simulink model "CANBlocksTemplate"  (Simulink 10.0)
settings: Solver=ode45  StartTime=0.0  StopTime=10.0  RelTol=1e-3  EnableMultiTasking=on
undefined symbols (not defined in the file): IO_Blk_Lib_TTC500, IO_Blk_Lib_TTC9094, IO_CAN_ConfigMsg, IO_CAN_Init, IO_CAN_ReadMsg
libraries: simulink x19, IOBlock_Library_TTC580 x18
(part 1 of 2)
settings Model: Creator=hokka  LastModifiedBy=hokka
settings Model: SuppressorTable=|
  | <?xml version="1.0" encoding="UTF-8" standalone="yes" ?>
  | <!DOCTYPE boost_serialization>
  | <boost_serialization signature="serialization::archive" version="15">
  | <DiagnosticSuppressor class_id="0" tracking_level="0" version="6">
  | 	<Table class_id="1" tracking_level="0" version="0">
  | 		<count>8</count>
  | 		<bucket_count>8</bucket_count>
  | 		<item_version>0</item_version>
  | 		<item class_id="2" tracking_level="0" version="0">
  | 			<first class_id="3" tracking_level="0" version="6">
  | 				<Source class_id="4" tracking_level="0" version="0">
  | 					<count>1</count>
  | 					<item_version>0</item_version>
  | 					<item>CANBlocksTemplate/CAN_RX_ND/Trigger_Block/Counter Limited</item>
  | 				</Source>
  | 			</first>
  | 			<second class_id="5" tracking_level="0" version="6">
  | 				<SuppressedData class_id="6" tracking_level="0" version="0">
  | 					<count>2</count>
  | 					<bucket_count>8</bucket_count>
  | 					<item_version>0</item_version>
  | 					<item class_id="7" tracking_level="0" version="0">
  | 						<first class_id="8" tracking_level="0" version="6">
  | 							<ID>SimulinkFixedPoint:util:Overflowoccurred</ID>
  | 							<Cause>
  | 								<Source>
  | 									<count>0</count>
  | 									<item_version>0</item_version>
  | 								</Source>
  | 							</Cause>
  | 						</first>
  | 						<second class_id="9" tracking_level="0" version="6">
  | 							<Comment></Comment>
  | 							<User></User>
  | 							<LastModified class_id="10" tracking_level="0" version="0">
  | 								<ptime_date class_id="11" tracking_level="0" version="0">
  | 									<date>20160608</date>
  | 								</ptime_date>
  | 								<ptime_time_duration class_id="12" tracking_level="0" version="0">
  | 									<is_special>0</is_special>
  | 									<time_duration_hours>15</time_duration_hours>
  | 									<time_duration_minutes>23</time_duration_minutes>
  | 									<time_duration_seconds>17</time_duration_seconds>
  | 									<time_duration_fractional_seconds>0</time_duration_fractional_seconds>
  | 								</ptime_time_duration>
  | 							</LastModified>
  | 							<SuppressionType>1</SuppressionType>
  | 						</second>
  | 					</item>
  | 					<item>
  | 						<first>
  | 							<ID>Simulink:DataType:WarningOverFlowDetected</ID>
  | 							<Cause>
  | 								<Source>
  | 									<count>0</count>
  | 									<item_version>0</item_version>
  | 								</Source>
  | 							</Cause>
  | 						</first>
  | 						<second>
  | 							<Comment></Comment>
  | 							<User></User>
  | 							<LastModified>
  | 								<ptime_date>
  | 									<date>20160608</date>
  | 								</ptime_date>
  | 								<ptime_time_duration>
  | 									<is_special>0</is_special>
  | 									<time_duration_hours>15</time_duration_hours>
  | 									<time_duration_minutes>23</time_duration_minutes>
  | 									<time_duration_seconds>17</time_duration_seconds>
  | 									<time_duration_fractional_seconds>0</time_duration_fractional_seconds>
  | 								</ptime_time_duration>
  | 							</LastModified>
  | 							<SuppressionType>1</SuppressionType>
  | 						</second>
  | 					</item>
  | 				</SuppressedData>
  | 			</second>
  | 		</item>
  | 		<item>
  | 			<first>
  | 				<Source>
  | 					<count>1</count>
  | 					<item_version>0</item_version>
  | 					<item>CANBlocksTemplate/CAN_TX/Trigger_Block/Counter Limited</item>
  | 				</Source>
  | 			</first>
  | 			<second>
  | 				<SuppressedData>
  | 					<count>2</count>
  | 					<bucket_count>8</bucket_count>
  | 					<item_version>0</item_version>
  | 					<item>
  | 						<first>
  | 							<ID>SimulinkFixedPoint:util:Overflowoccurred</ID>
  | 							<Cause>
  | 								<Source>
  | 									<count>0</count>
  | 									<item_version>0</item_version>
  | 								</Source>
  | 							</Cause>
  | 						</first>
  | 						<second>
  | 							<Comment></Comment>
  | 							<User></User>
  | 							<LastModified>
  | 								<ptime_date>
  | 									<date>20160608</date>
  | 								</ptime_date>
  | 								<ptime_time_duration>
  | 									<is_special>0</is_special>
  | 									<time_duration_hours>15</time_duration_hours>
  | 									<time_duration_minutes>23</time_duration_minutes>
  | 									<time_duration_seconds>17</time_duration_seconds>
  | 									<time_duration_fractional_seconds>0</time_duration_fractional_seconds>
  | 								</ptime_time_duration>
  | 							</LastModified>
  | 							<SuppressionType>1</SuppressionType>
  | 						</second>
  | 					</item>
  | 					<item>
  | 						<first>
  | 							<ID>Simulink:DataType:WarningOverFlowDetected</ID>
  | 							<Cause>
  | 								<Source>
  | 									<count>0</count>
  | 									<item_version>0</item_version>
  | 								</Source>
  | 							</Cause>
  | 						</first>
  | 						<second>
  | 							<Comment></Comment>
  | 							<User></User>
  | 							<LastModified>
  | 								<ptime_date>
  | 									<date>20160608</date>
  | 								</ptime_date>
  | 								<ptime_time_duration>
  | 									<is_special>0</is_special>
  | 									<time_duration_hours>15</time_duration_hours>
  | 									<time_duration_minutes>23</time_duration_minutes>
  | 									<time_duration_seconds>17</time_duration_seconds>
  | 									<time_duration_fractional_seconds>0</time_duration_fractional_seconds>
  | 								</ptime_time_duration>
  | 							</LastModified>
  | 							<SuppressionType>1</SuppressionType>
  | 						</second>
  | 					</item>
  | 				</SuppressedData>
  | 			</second>
  | 		</item>
  | 		<item>
  | 			<first>
  | 				<Source>
  | 					<count>1</count>
  | 					<item_version>0</item_version>
  | 					<item>CANBlocksTemplate/CAN_RX_NONE_ND/Trigger_Block/Counter Limited</item>
  | 				</Source>
  | 			</first>
  | 			<second>
  | 				<SuppressedData>
  | 					<count>2</count>
  | 					<bucket_count>8</bucket_count>
  | 					<item_version>0</item_version>
  | 					<item>
  | 						<first>
  | 							<ID>SimulinkFixedPoint:util:Overflowoccurred</ID>
  | 							<Cause>
  | 								<Source>
  | 									<count>0</count>
  | 									<item_version>0</item_version>
  | 								</Source>
  | 							</Cause>
  | 						</first>
  | 						<second>
  | 							<Comment></Comment>
  | 							<User></User>
  | 							<LastModified>
  | 								<ptime_date>
  | 									<date>20160608</date>
  | 								</ptime_date>
  | 								<ptime_time_duration>
  | 									<is_special>0</is_special>
  | 									<time_duration_hours>15</time_duration_hours>
  | 									<time_duration_minutes>23</time_duration_minutes>
  | 									<time_duration_seconds>17</time_duration_seconds>
  | 									<time_duration_fractional_seconds>0</time_duration_fractional_seconds>
  | 								</ptime_time_duration>
  | 							</LastModified>
  | 							<SuppressionType>1</SuppressionType>
  | 						</second>
  | 					</item>
  | 					<item>
  | 						<first>
  | 							<ID>Simulink:DataType:WarningOverFlowDetected</ID>
  | 							<Cause>
  | 								<Source>
  | 									<count>0</count>
  | 									<item_version>0</item_version>
  | 								</Source>
  | 							</Cause>
  | 						</first>
  | 						<second>
  | 							<Comment></Comment>
  | 							<User></User>
  | 							<LastModified>
  | 								<ptime_date>
  | 									<date>20160608</date>
  | 								</ptime_date>
  | 								<ptime_time_duration>
  | 									<is_special>0</is_special>
  | 									<time_duration_hours>15</time_duration_hours>
  | 									<time_duration_minutes>23</time_duration_minutes>
  | 									<time_duration_seconds>17</time_duration_seconds>
  | 									<time_duration_fractional_seconds>0</time_duration_fractional_seconds>
  | 								</ptime_time_duration>
  | 							</LastModified>
  | 							<SuppressionType>1</SuppressionType>
  | 						</second>
  | 					</item>
  | 				</SuppressedData>
  | 			</second>
  | 		</item>
  | 		<item>
  | 			<first>
  | 				<Source>
  | 					<count>1</count>
  | 					<item_version>0</item_version>
  | 					<item>CANBlocksTemplate/CAN_TX_NONE_aggr/Trigger_Block/Counter Limited</item>
  | 				</Source>
  | 			</first>
  | 			<second>
  | 				<SuppressedData>
  | 					<count>2</count>
  | 					<bucket_count>8</bucket_count>
  | 					<item_version>0</item_version>
  | 					<item>
  | 						<first>
  | 							<ID>SimulinkFixedPoint:util:Overflowoccurred</ID>
  | 							<Cause>
  | 								<Source>
  | 									<count>0</count>
  | 									<item_version>0</item_version>
  | 								</Source>
  | 							</Cause>
  | 						</first>
  | 						<second>
  | 							<Comment></Comment>
  | 							<User></User>
  | 							<LastModified>
  | 								<ptime_date>
  | 									<date>20160608</date>
  | 								</ptime_date>
  | 								<ptime_time_duration>
  | 									<is_special>0</is_special>
  | 									<time_duration_hours>15</time_duration_hours>
  | 									<time_duration_minutes>23</time_duration_minutes>
  | 									<time_duration_seconds>17</time_duration_seconds>
  | 									<time_duration_fractional_seconds>0</time_duration_fractional_seconds>
  | 								</ptime_time_duration>
  | 							</LastModified>
  | 							<SuppressionType>1</SuppressionType>
  | 						</second>
  | 					</item>
  | 					<item>
  | 						<first>
  | 							<ID>Simulink:DataType:WarningOverFlowDetected</ID>
  | 							<Cause>
  | 								<Source>
  | 									<count>0</count>
  | 									<item_version>0</item_version>
  | 								</Source>
  | 							</Cause>
  | 						</first>
  | 						<second>
  | 							<Comment></Comment>
  | 							<User></User>
  | 							<LastModified>
  | 								<ptime_date>
  | 									<date>20160608</date>
  | 								</ptime_date>
  | 								<ptime_time_duration>
  | 									<is_special>0</is_special>
  | 									<time_duration_hours>15</time_duration_hours>
  | 									<time_duration_minutes>23</time_duration_minutes>
  | 									<time_duration_seconds>17</time_duration_seconds>
  | 									<time_duration_fractional_seconds>0</time_duration_fractional_seconds>
  | 								</ptime_time_duration>
  | 							</LastModified>
  | 							<SuppressionType>1</SuppressionType>
  | 						</second>
  | 					</item>
  | 				</SuppressedData>
  | 			</second>
  | 		</item>
  | 		<item>
  | 			<first>
  | 				<Source>
  | 					<count>1</count>
  | 					<item_version>0</item_version>
  | 					<item>CANBlocksTemplate/CAN_TX_NONE/Trigger_Block/Counter Limited</item>
  | 				</Source>
  | 			</first>
  | 			<second>
  | 				<SuppressedData>
  | 					<count>2</count>
  | 					<bucket_count>8</bucket_count>
  | 					<item_version>0</item_version>
  | 					<item>
  | 						<first>
  | 							<ID>SimulinkFixedPoint:util:Overflowoccurred</ID>
  | 							<Cause>
  | 								<Source>
  | 									<count>0</count>
  | 									<item_version>0</item_version>
  | 								</Source>
  | 							</Cause>
  | 						</first>
  | 						<second>
  | 							<Comment></Comment>
  | 							<User></User>
  | 							<LastModified>
  | 								<ptime_date>
  | 									<date>20160608</date>
  | 								</ptime_date>
  | 								<ptime_time_duration>
  | 									<is_special>0</is_special>
  | 									<time_duration_hours>15</time_duration_hours>
  | 									<time_duration_minutes>23</time_duration_minutes>
  | 									<time_duration_seconds>17</time_duration_seconds>
  | 									<time_duration_fractional_seconds>0</time_duration_fractional_seconds>
  | 								</ptime_time_duration>
  | 							</LastModified>
  | 							<SuppressionType>1</SuppressionType>
  | 						</second>
  | 					</item>
  | 					<item>
  | 						<first>
  | 							<ID>Simulink:DataType:WarningOverFlowDetected</ID>
  | 							<Cause>
  | 								<Source>
  | 									<count>0</count>
  | 									<item_version>0</item_version>
  | 								</Source>
  | 							</Cause>
  | 						</first>
  | 						<second>
  | 							<Comment></Comment>
  | 							<User></User>
  | 							<LastModified>
  | 								<ptime_date>
  | 									<date>20160608</date>
  | 								</ptime_date>
  | 								<ptime_time_duration>
  | 									<is_special>0</is_special>
  | 									<time_duration_hours>15</time_duration_hours>
  | 									<time_duration_minutes>23</time_duration_minutes>
  | 									<time_duration_seconds>17</time_duration_seconds>
  | 									<time_duration_fractional_seconds>0</time_duration_fractional_seconds>
  | 								</ptime_time_duration>
  | 							</LastModified>
  | 							<SuppressionType>1</SuppressionType>
  | 						</second>
  | 					</item>
  | 				</SuppressedData>
  | 			</second>
  | 		</item>
  | 		<item>
  | 			<first>
  | 				<Source>
  | 					<count>1</count>
  | 					<item_version>0</item_version>
  | 					<item>CANBlocksTemplate/CAN_RX/Trigger_Block/Counter Limited</item>
  | 				</Source>
  | 			</first>
  | 			<second>
  | 				<SuppressedData>
  | 					<count>2</count>
  | 					<bucket_count>8</bucket_count>
  | 					<item_version>0</item_version>
  | 					<item>
  | 						<first>
  | 							<ID>SimulinkFixedPoint:util:Overflowoccurred</ID>
  | 							<Cause>
  | 								<Source>
  | 									<count>0</count>
  | 									<item_version>0</item_version>
  | 								</Source>
  | 							</Cause>
  | 						</first>
  | 						<second>
  | 							<Comment></Comment>
  | 							<User></User>
  | 							<LastModified>
  | 								<ptime_date>
  | 									<date>20160608</date>
  | 								</ptime_date>
  | 								<ptime_time_duration>
  | 									<is_special>0</is_special>
  | 									<time_duration_hours>15</time_duration_hours>
  | 									<time_duration_minutes>23</time_duration_minutes>
  | 									<time_duration_seconds>17</time_duration_seconds>
  | 									<time_duration_fractional_seconds>0</time_duration_fractional_seconds>
  | 								</ptime_time_duration>
  | 							</LastModified>
  | 							<SuppressionType>1</SuppressionType>
  | 						</second>
  | 					</item>
  | 					<item>
  | 						<first>
  | 							<ID>Simulink:DataType:WarningOverFlowDetected</ID>
  | 							<Cause>
  | 								<Source>
  | 									<count>0</count>
  | 									<item_version>0</item_version>
  | 								</Source>
  | 							</Cause>
  | 						</first>
  | 						<second>
  | 							<Comment></Comment>
  | 							<User></User>
  | 							<LastModified>
  | 								<ptime_date>
  | 									<date>20160608</date>
  | 								</ptime_date>
  | 								<ptime_time_duration>
  | 									<is_special>0</is_special>
  | 									<time_duration_hours>15</time_duration_hours>
  | 									<time_duration_minutes>23</time_duration_minutes>
  | 									<time_duration_seconds>17</time_duration_seconds>
  | 									<time_duration_fractional_seconds>0</time_duration_fractional_seconds>
  | 								</ptime_time_duration>
  | 							</LastModified>
  | 							<SuppressionType>1</SuppressionType>
  | 						</second>
  | 					</item>
  | 				</SuppressedData>
  | 			</second>
  | 		</item>
  | 		<item>
  | 			<first>
  | 				<Source>
  | 					<count>1</count>
  | 					<item_version>0</item_version>
  | 					<item>CANBlocksTemplate/CAN_RX_NONE/Trigger_Block/Counter Limited</item>
  | 				</Source>
  | 			</first>
  | 			<second>
  | 				<SuppressedData>
  | 					<count>2</count>
  | 					<bucket_count>8</bucket_count>
  | 					<item_version>0</item_version>
  | 					<item>
  | 						<first>
  | 							<ID>SimulinkFixedPoint:util:Overflowoccurred</ID>
  | 							<Cause>
  | 								<Source>
  | 									<count>0</count>
  | 									<item_version>0</item_version>
  | 								</Source>
  | 							</Cause>
  | 						</first>
  | 						<second>
  | 							<Comment></Comment>
  | 							<User></User>
  | 							<LastModified>
  | 								<ptime_date>
  | 									<date>20160608</date>
  | 								</ptime_date>
  | 								<ptime_time_duration>
  | 									<is_special>0</is_special>
  | 									<time_duration_hours>15</time_duration_hours>
  | 									<time_duration_minutes>23</time_duration_minutes>
  | 									<time_duration_seconds>17</time_duration_seconds>
  | 									<time_duration_fractional_seconds>0</time_duration_fractional_seconds>
  | 								</ptime_time_duration>
  | 							</LastModified>
  | 							<SuppressionType>1</SuppressionType>
  | 						</second>
  | 					</item>
  | 					<item>
  | 						<first>
  | 							<ID>Simulink:DataType:WarningOverFlowDetected</ID>
  | 							<Cause>
  | 								<Source>
  | 									<count>0</count>
  | 									<item_version>0</item_version>
  | 								</Source>
  | 							</Cause>
  | 						</first>
  | 						<second>
  | 							<Comment></Comment>
  | 							<User></User>
  | 							<LastModified>
  | 								<ptime_date>
  | 									<date>20160608</date>
  | 								</ptime_date>
  | 								<ptime_time_duration>
  | 									<is_special>0</is_special>
  | 									<time_duration_hours>15</time_duration_hours>
  | 									<time_duration_minutes>23</time_duration_minutes>
  | 									<time_duration_seconds>17</time_duration_seconds>
  | 									<time_duration_fractional_seconds>0</time_duration_fractional_seconds>
  | 								</ptime_time_duration>
  | 							</LastModified>
  | 							<SuppressionType>1</SuppressionType>
  | 						</second>
  | 					</item>
  | 				</SuppressedData>
  | 			</second>
  | 		</item>
  | 		<item>
  | 			<first>
  | 				<Source>
  | 					<count>1</count>
  | 					<item_version>0</item_version>
  | 					<item>CANBlocksTemplate/CAN_TX_aggr/Trigger_Block/Counter Limited</item>
  | 				</Source>
  | 			</first>
  | 			<second>
  | 				<SuppressedData>
  | 					<count>2</count>
  | 					<bucket_count>8</bucket_count>
  | 					<item_version>0</item_version>
  | 					<item>
  | 						<first>
  | 							<ID>Simulink:DataType:WarningOverFlowDetected</ID>
  | 							<Cause>
  | 								<Source>
  | 									<count>0</count>
  | 									<item_version>0</item_version>
  | 								</Source>
  | 							</Cause>
  | 						</first>
  | 						<second>
  | 							<Comment></Comment>
  | 							<User></User>
  | 							<LastModified>
  | 								<ptime_date>
  | 									<date>20160608</date>
  | 								</ptime_date>
  | 								<ptime_time_duration>
  | 									<is_special>0</is_special>
  | 									<time_duration_hours>15</time_duration_hours>
  | 									<time_duration_minutes>23</time_duration_minutes>
  | 									<time_duration_seconds>17</time_duration_seconds>
  | 									<time_duration_fractional_seconds>0</time_duration_fractional_seconds>
  | 								</ptime_time_duration>
  | 							</LastModified>
  | 							<SuppressionType>1</SuppressionType>
  | 						</second>
  | 					</item>
  | 					<item>
  | 						<first>
  | 							<ID>SimulinkFixedPoint:util:Overflowoccurred</ID>
  | 							<Cause>
  | 								<Source>
  | 									<count>0</count>
  | 									<item_version>0</item_version>
  | 								</Source>
  | 							</Cause>
  | 						</first>
  | 						<second>
  | 							<Comment></Comment>
  | 							<User></User>
  | 							<LastModified>
  | 								<ptime_date>
  | 									<date>20160608</date>
  | 								</ptime_date>
  | 								<ptime_time_duration>
  | 									<is_special>0</is_special>
  | 									<time_duration_hours>15</time_duration_hours>
  | 									<time_duration_minutes>23</time_duration_minutes>
  | 									<time_duration_seconds>17</time_duration_seconds>
  | 									<time_duration_fractional_seconds>0</time_duration_fractional_seconds>
  | 								</ptime_time_duration>
  | 							</LastModified>
  | 							<SuppressionType>1</SuppressionType>
  | 						</second>
  | 					</item>
  | 				</SuppressedData>
  | 			</second>
  | 		</item>
  | 	</Table>
  | </DiagnosticSuppressor>
  | </boost_serialization>
settings DataIOCC: LimitDataPoints=on  SignalLoggingSaveFormat=ModelDataLogs
settings OptimizationCC: ExpressionDepthLimit=2147483647
settings DebuggingCC: SolverPrmCheckMsg=warning  FcnCallInpInsideContextMsg=warning  StateNameClashWarn=warning
settings ConfigComp: CovExternalEMLEnable=off

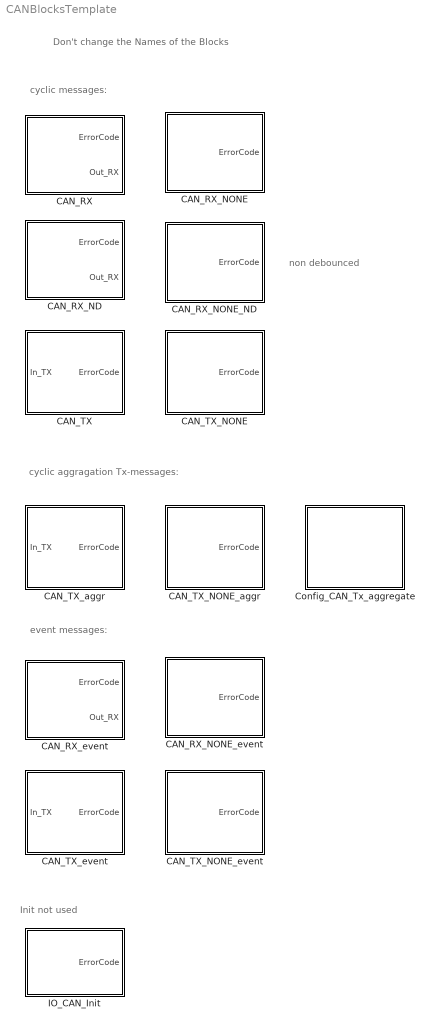
== system CANBlocksTemplate ==
  note: Don't change the Names of the Blocks
  note: cyclic messages:
  note: event messages:
  note: Init not used
  note: non debounced
  note: cyclic aggragation Tx-messages:
  CAN_RX : Subsystem  Priority=0
  CAN_RX_ND : Subsystem  Priority=0
  CAN_RX_NONE : Subsystem  Priority=0
  CAN_RX_NONE_ND : Subsystem  Priority=0
  CAN_RX_NONE_event : Subsystem  Priority=0
  CAN_RX_event : Subsystem  Priority=0
  CAN_TX : Subsystem  Priority=0
  CAN_TX_NONE : Subsystem  Priority=0
  CAN_TX_NONE_aggr : Subsystem  Priority=0  mask(CAN block for aggregated Tx messages){CANChannel_TopMask=0, CycleTime_TopMask=0, Offset_TopMask=0}
      mask prompts: CANChannel_TopMask "CAN channel"; CycleTime_TopMask "CycleTime [ms]"; Offset_TopMask "Offset [ms]"
      mask help: Drag this Block into the model to define an aggregated CAN Tx-message.
      mask Help:
      | Drag this Block into the model to define the handle for aggregated CAN Tx-messages
      | Aggregated CAN Tx-messages with the same cycle time are sent out sequentially sharing a common message object.
      | This given aggregated CAN-Tx block needs the corresponding "Tx-CAN Config Master"-block to reside in the same model.  If not, an ErrorCode for missing handle  is issued during execution on the target.
      | 
      | Mask information entries (not for configuration purposes):
      | CAN channel: The message is sent out over the given channel number
      | CycleTime [ms]: The message is repetitively sent out with the given cycle time.
      | Offset [ms]: Within the sequence of repetative CAN messages, the sequence position of the message is defined by the given offset.
      | 
      | In order to provide reduced amount of handles the DBC_Importer can be configured to collect CAN Tx-messages with high cycle times to be processed by single message objects. By doing so the application saves the limited amount of CAN message objects in favor of higher frequency CAN Tx-messages and the event messages.
      | 
      | Limitation: The generated CAN Tx-message blocks are squentially transmitted over the specified CAN channel. The sequence cannot be defined beforehand.
  CAN_TX_NONE_event : Subsystem  Priority=0
  CAN_TX_aggr : Subsystem  Priority=0  mask(CAN block for aggregated Tx messages){CANChannel_TopMask=0, CycleTime_TopMask=0, Offset_TopMask=0}
      mask prompts: CANChannel_TopMask "CAN channel"; CycleTime_TopMask "CycleTime [ms]"; Offset_TopMask "Offset [ms]"
      mask help: Drag this Block into the model to define an aggregated CAN Tx-message.
      mask Help:
      | Drag this Block into the model to define the handle for aggregated CAN Tx-messages
      | Aggregated CAN Tx-messages with the same cycle time are sent out sequentially sharing a common message object.
      | This given aggregated CAN-Tx block needs the corresponding "Tx-CAN Config Master"-block to reside in the same model. If not, an ErrorCode for missing handle  is issued during execution on the target.
      | 
      | Mask information entries (not for configuration purposes)
      | CAN channel: The message is sent out over the given channel number
      | CycleTime [ms]: The message is repetitively sent out with the given cycle time.
      | Offset [ms]: Within the sequence of repetative CAN messages, the sequence position of the message is defined by the given offset.
      | 
      | In order to provide reduced amount of handles the DBC_Importer can be configured to collect CAN Tx-messages with high cycle times to be processed by single message objects. By doing so the application saves the limited amount of CAN message objects in favor of higher frequency CAN Tx-messages and the event messages.
      | 
      | Limitation: The generated CAN Tx-message blocks are squentially transmitted over the specified CAN channel. The sequence cannot be defined beforehand.
  CAN_TX_event : Subsystem  Priority=0
  Config_CAN_Tx_aggregate : Subsystem  Priority=0  mask(CAN Config for aggregated Tx messages){}
      mask help: Drag this Block into the model to define the handle for aggregated CAN Tx-messages
      mask Help:
      | This block is generated automatically by DBC_Import of the IOLib.
      | 
      | In order to provide reduced amount of handles the DBC_Importer can be configured to collect CAN Tx-messages with high cycle times to be processed by single message objects. By doing so the application saves the limited amount of CAN message objects in favor of higher frequency CAN Tx-messages and the event messages.
      | Aggregated CAN-Tx block need to reside in the same model together with this corresponding "Tx-CAN Config Master"-block.  If not, an ErrorCode for missing handle  is issued by the respective CAN-Tx call during execution on the target.
      | 
      | Limitation: The generated CAN Tx-message blocks are squentially transmitted over the specified CAN channel. The sequence cannot be defined beforehand.
      mask Display: disp('<tbd>')
  IO_CAN_Init : Subsystem  Priority=-2147483646  mask(IO_CAN_Init_Code){SampleTime=-1, ttlib=IO_Blk_Lib_TTC9094, ttDescription=IO_CAN_Init, tt_iolib_version=0.19, channel=IO_CAN_CHANNEL_0, baudrate=500, tseg1=5, tseg2=3, sjw=2}
      mask help: Representation of the IO_CAN_Init function call
      settings: CopyFcn=set_param(gcbh, 'LinkStatus', 'none')
      mask Help: web(which('IO_CAN.h'))
      mask TypeOptions channel: IO_CAN_CHANNEL_0  | IO_CAN_CHANNEL_1 | IO_CAN_CHANNEL_2 | IO_CAN_CHANNEL_3
      mask TypeOptions baudrate: 10 | 20 | 50 | 100 | 125 | 250 | 500 | 1000
      mask TypeOptions tseg1: 3 | 4 | 5 | 6 | 7 | 8 | 9 | 10 | 11 | 12 | 13 | 14 | 15 | 16
      mask TypeOptions tseg2: 2 | 3 | 4 | 5 | 6 | 7 | 8
      mask TypeOptions sjw: 1 | 2 | 3 | 4
      mask Display: disp('NOT USED TTC580')

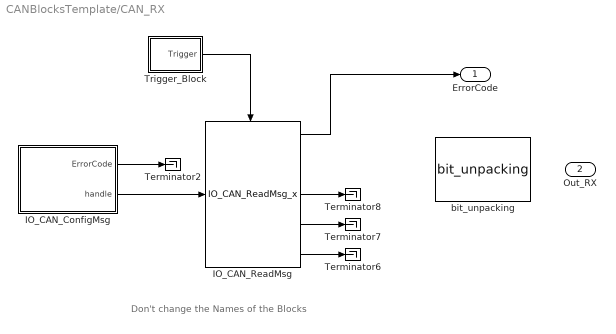
== system CANBlocksTemplate/CAN_RX ==
  note: Don't change the Names of the Blocks
  IO_CAN_ConfigMsg : Subsystem  mask(IO_CAN_ConfigMsg_Code){SampleTime=-1, ttlib=IO_Blk_Lib_TTC500, ttDescription=IO_CAN_ConfigMsg, tt_iolib_version=0.19, channel=IO_CAN_CHANNEL_0, mode=IO_CAN_MSG_READ, id_format=IO_CAN_STD_FRAME, id=0x1, ac_mask=0x7FF}
      mask help: Configures a message object for the given CAN channel.
      mask init:
      | %
      settings: CopyFcn=%deleted
      mask Help: web(which('IO_CAN.h'))
      mask TypeOptions channel: IO_CAN_CHANNEL_0  | IO_CAN_CHANNEL_1 | IO_CAN_CHANNEL_2 | IO_CAN_CHANNEL_3 | IO_CAN_CHANNEL_4 | IO_CAN_CHANNEL_5 | IO_CAN_CHANNEL_6
      mask Callback channel: %
      mask TypeOptions mode: IO_CAN_MSG_READ | IO_CAN_MSG_WRITE
      mask Callback mode: %
      mask TypeOptions id_format: IO_CAN_STD_FRAME | IO_CAN_EXT_FRAME
      mask Callback id_format: %
      mask Callback id: %
      mask Callback ac_mask: %
  IO_CAN_ReadMsg : IOBlock_Library_TTC580/CAN  Blocks TTC580 IOlib/ReadMsg_CAN_derated/IO_CAN_ReadMsg_x  SampleTime=-1  ttlib=IO_Blk_Lib_TTC500  ttDescription=IO_CAN_ReadMsg  tt_iolib_version=0.19
      settings: SourceProductName=I/O Blocklibrary for TTC580
  Terminator{2,6..8} (4 alike) : Terminator
  Trigger_Block : Subsystem  mask(Derate Trigger){derate=1, trigger_offset=0}
      mask prompts: trigger_offset "offset for the trigger"
      mask help: derate "n": every n-th cylce a trigger is submitted
  bit_unpacking : IOBlock_Library_TTC580/CAN  Blocks TTC580 IOlib/bit_unpacking  SampleTime=-1  ttlib=IO_Blk_Lib_TTC500  ttDescription=bit_unpacking  tt_iolib_version=0.26  Endianness=little  Format=unsigned  Inversion=off  Startbit=0  Width_bits=8  Factor=1.0  Offset=0.0
      settings: SourceProductName=I/O Blocklibrary for TTC580
  ErrorCode : Outport  VectorParamsAs1DForOutWhenUnconnected=off
  Out_RX : Outport  Port=2  VectorParamsAs1DForOutWhenUnconnected=off
  wires:
  IO_CAN_ReadMsg/3 -> Terminator8/1
  IO_CAN_ReadMsg/4 -> Terminator7/1
  IO_CAN_ReadMsg/5 -> Terminator6/1
  IO_CAN_ConfigMsg/2(handle) -> IO_CAN_ReadMsg/1
  IO_CAN_ConfigMsg/1(ErrorCode) -> Terminator2/1
  Trigger_Block/1(Trigger) -> IO_CAN_ReadMsg/Enable
  IO_CAN_ReadMsg/1 -> ErrorCode/1

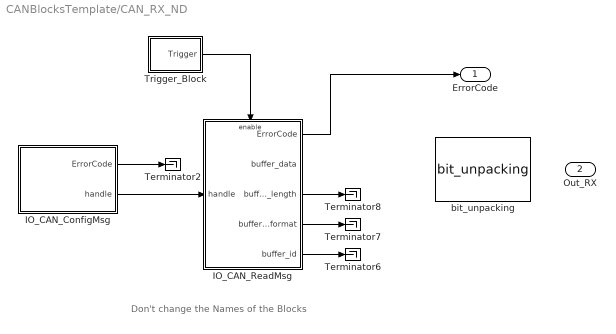
== system CANBlocksTemplate/CAN_RX_ND ==
  note: Don't change the Names of the Blocks
  IO_CAN_ConfigMsg : Subsystem  mask(IO_CAN_ConfigMsg_Code){SampleTime=-1, ttlib=IO_Blk_Lib_TTC500, ttDescription=IO_CAN_ConfigMsg, tt_iolib_version=0.19, channel=IO_CAN_CHANNEL_0, mode=IO_CAN_MSG_READ, id_format=IO_CAN_STD_FRAME, id=0x1, ac_mask=0x7FF}
      mask help: Configures a message object for the given CAN channel.
      mask init:
      | %
      settings: CopyFcn=%deleted
      mask Help: web(which('IO_CAN.h'))
      mask TypeOptions channel: IO_CAN_CHANNEL_0  | IO_CAN_CHANNEL_1 | IO_CAN_CHANNEL_2 | IO_CAN_CHANNEL_3 | IO_CAN_CHANNEL_4 | IO_CAN_CHANNEL_5 | IO_CAN_CHANNEL_6
      mask Callback channel: %
      mask TypeOptions mode: IO_CAN_MSG_READ | IO_CAN_MSG_WRITE
      mask Callback mode: %
      mask TypeOptions id_format: IO_CAN_STD_FRAME | IO_CAN_EXT_FRAME
      mask Callback id_format: %
      mask Callback id: %
      mask Callback ac_mask: %
  IO_CAN_ReadMsg : Subsystem  mask(IO_CAN_ReadMsg_Code){SampleTime=-1, ttlib=IO_Blk_Lib_TTC500, ttDescription=IO_CAN_ReadMsg, tt_iolib_version=0.19}
      mask help: Reads a message from a given message object.
      mask init:
      | %
      settings: CopyFcn=%deleted
      mask Help: web(which('IO_CAN.h'))
  Terminator{2,6..8} (4 alike) : Terminator
  Trigger_Block : Subsystem  mask(Derate Trigger){derate=1, trigger_offset=0}
      mask prompts: trigger_offset "offset for the trigger"
      mask help: derate "n": every n-th cylce a trigger is submitted
  bit_unpacking : IOBlock_Library_TTC580/CAN  Blocks TTC580 IOlib/bit_unpacking  SampleTime=-1  ttlib=IO_Blk_Lib_TTC500  ttDescription=bit_unpacking  tt_iolib_version=0.26  Endianness=little  Format=unsigned  Inversion=off  Startbit=0  Width_bits=8  Factor=1.0  Offset=0.0
      settings: SourceProductName=I/O Blocklibrary for TTC580
  ErrorCode : Outport  VectorParamsAs1DForOutWhenUnconnected=off
  Out_RX : Outport  Port=2  VectorParamsAs1DForOutWhenUnconnected=off
  wires:
  IO_CAN_ReadMsg/1(ErrorCode) -> ErrorCode/1
  Trigger_Block/1(Trigger) -> IO_CAN_ReadMsg/Enable
  IO_CAN_ConfigMsg/1(ErrorCode) -> Terminator2/1
  IO_CAN_ConfigMsg/2(handle) -> IO_CAN_ReadMsg/1(handle)
  IO_CAN_ReadMsg/5(buffer_id) -> Terminator6/1
  IO_CAN_ReadMsg/4(buffer_id_format) -> Terminator7/1
  IO_CAN_ReadMsg/3(buffer_length) -> Terminator8/1

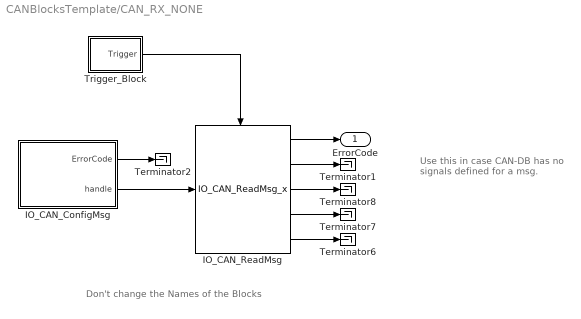
== system CANBlocksTemplate/CAN_RX_NONE ==
  note: Use this in case CAN-DB
      | has no signals defined for a msg.
  note: Don't change the Names of the Blocks
  IO_CAN_ConfigMsg : Subsystem  mask(IO_CAN_ConfigMsg_Code){SampleTime=-1, ttlib=IO_Blk_Lib_TTC500, ttDescription=IO_CAN_ConfigMsg, tt_iolib_version=0.19, channel=IO_CAN_CHANNEL_0, mode=IO_CAN_MSG_READ, id_format=IO_CAN_STD_FRAME, id=0x1, ac_mask=0x7FF}
      mask help: Configures a message object for the given CAN channel.
      mask init:
      | %
      settings: CopyFcn=%deleted
      mask Help: web(which('IO_CAN.h'))
      mask TypeOptions channel: IO_CAN_CHANNEL_0  | IO_CAN_CHANNEL_1 | IO_CAN_CHANNEL_2 | IO_CAN_CHANNEL_3 | IO_CAN_CHANNEL_4 | IO_CAN_CHANNEL_5 | IO_CAN_CHANNEL_6
      mask Callback channel: %
      mask TypeOptions mode: IO_CAN_MSG_READ | IO_CAN_MSG_WRITE
      mask Callback mode: %
      mask TypeOptions id_format: IO_CAN_STD_FRAME | IO_CAN_EXT_FRAME
      mask Callback id_format: %
      mask Callback id: %
      mask Callback ac_mask: %
  IO_CAN_ReadMsg : IOBlock_Library_TTC580/CAN  Blocks TTC580 IOlib/ReadMsg_CAN_derated/IO_CAN_ReadMsg_x  SampleTime=-1  ttlib=IO_Blk_Lib_TTC500  ttDescription=IO_CAN_ReadMsg  tt_iolib_version=0.19
      settings: SourceProductName=I/O Blocklibrary for TTC580
  Terminator{1..2,6..8} (5 alike) : Terminator
  Trigger_Block : Subsystem  mask(Derate Trigger){derate=1, trigger_offset=0}
      mask prompts: trigger_offset "offset for the trigger"
      mask help: derate "n": every n-th cylce a trigger is submitted
  ErrorCode : Outport  VectorParamsAs1DForOutWhenUnconnected=off
  wires:
  IO_CAN_ReadMsg/3 -> Terminator8/1
  IO_CAN_ReadMsg/4 -> Terminator7/1
  IO_CAN_ReadMsg/5 -> Terminator6/1
  IO_CAN_ReadMsg/1 -> ErrorCode/1
  IO_CAN_ReadMsg/2 -> Terminator1/1
  IO_CAN_ConfigMsg/2(handle) -> IO_CAN_ReadMsg/1
  IO_CAN_ConfigMsg/1(ErrorCode) -> Terminator2/1
  Trigger_Block/1(Trigger) -> IO_CAN_ReadMsg/Enable

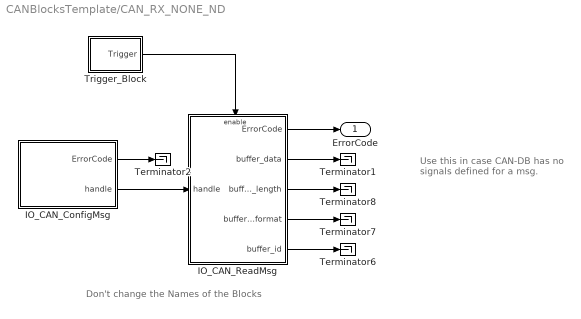
== system CANBlocksTemplate/CAN_RX_NONE_ND ==
  note: Don't change the Names of the Blocks
  note: Use this in case CAN-DB
      | has no signals defined for a msg.
  IO_CAN_ConfigMsg : Subsystem  mask(IO_CAN_ConfigMsg_Code){SampleTime=-1, ttlib=IO_Blk_Lib_TTC500, ttDescription=IO_CAN_ConfigMsg, tt_iolib_version=0.19, channel=IO_CAN_CHANNEL_0, mode=IO_CAN_MSG_READ, id_format=IO_CAN_STD_FRAME, id=0x1, ac_mask=0x7FF}
      mask help: Configures a message object for the given CAN channel.
      mask init:
      | %
      settings: CopyFcn=%deleted
      mask Help: web(which('IO_CAN.h'))
      mask TypeOptions channel: IO_CAN_CHANNEL_0  | IO_CAN_CHANNEL_1 | IO_CAN_CHANNEL_2 | IO_CAN_CHANNEL_3 | IO_CAN_CHANNEL_4 | IO_CAN_CHANNEL_5 | IO_CAN_CHANNEL_6
      mask Callback channel: %
      mask TypeOptions mode: IO_CAN_MSG_READ | IO_CAN_MSG_WRITE
      mask Callback mode: %
      mask TypeOptions id_format: IO_CAN_STD_FRAME | IO_CAN_EXT_FRAME
      mask Callback id_format: %
      mask Callback id: %
      mask Callback ac_mask: %
  IO_CAN_ReadMsg : Subsystem  mask(IO_CAN_ReadMsg_Code){SampleTime=-1, ttlib=IO_Blk_Lib_TTC500, ttDescription=IO_CAN_ReadMsg, tt_iolib_version=0.19}
      mask help: Reads a message from a given message object.
      mask init:
      | %
      settings: CopyFcn=%deleted
      mask Help: web(which('IO_CAN.h'))
  Terminator{1..2,6..8} (5 alike) : Terminator
  Trigger_Block : Subsystem  mask(Derate Trigger){derate=1, trigger_offset=0}
      mask prompts: trigger_offset "offset for the trigger"
      mask help: derate "n": every n-th cylce a trigger is submitted
  ErrorCode : Outport  VectorParamsAs1DForOutWhenUnconnected=off
  wires:
  Trigger_Block/1(Trigger) -> IO_CAN_ReadMsg/Enable
  IO_CAN_ConfigMsg/1(ErrorCode) -> Terminator2/1
  IO_CAN_ConfigMsg/2(handle) -> IO_CAN_ReadMsg/1(handle)
  IO_CAN_ReadMsg/2(buffer_data) -> Terminator1/1
  IO_CAN_ReadMsg/1(ErrorCode) -> ErrorCode/1
  IO_CAN_ReadMsg/5(buffer_id) -> Terminator6/1
  IO_CAN_ReadMsg/4(buffer_id_format) -> Terminator7/1
  IO_CAN_ReadMsg/3(buffer_length) -> Terminator8/1

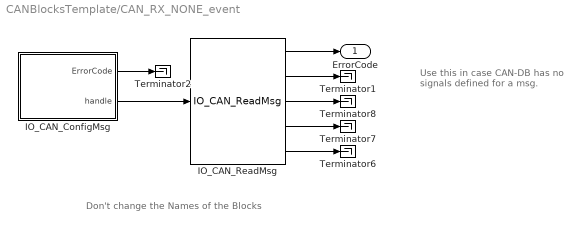
== system CANBlocksTemplate/CAN_RX_NONE_event ==
  note: Don't change the Names of the Blocks
  note: Use this in case CAN-DB
      | has no signals defined for a msg.
  IO_CAN_ConfigMsg : Subsystem  mask(IO_CAN_ConfigMsg_Code){SampleTime=-1, ttlib=IO_Blk_Lib_TTC500, ttDescription=IO_CAN_ConfigMsg, tt_iolib_version=0.19, channel=IO_CAN_CHANNEL_0, mode=IO_CAN_MSG_READ, id_format=IO_CAN_STD_FRAME, id=0x1, ac_mask=0x7FF}
      mask help: Configures a message object for the given CAN channel.
      mask init:
      | %
      settings: CopyFcn=%deleted
      mask Help: web(which('IO_CAN.h'))
      mask TypeOptions channel: IO_CAN_CHANNEL_0  | IO_CAN_CHANNEL_1 | IO_CAN_CHANNEL_2 | IO_CAN_CHANNEL_3 | IO_CAN_CHANNEL_4 | IO_CAN_CHANNEL_5 | IO_CAN_CHANNEL_6
      mask Callback channel: %
      mask TypeOptions mode: IO_CAN_MSG_READ | IO_CAN_MSG_WRITE
      mask Callback mode: %
      mask TypeOptions id_format: IO_CAN_STD_FRAME | IO_CAN_EXT_FRAME
      mask Callback id_format: %
      mask Callback id: %
      mask Callback ac_mask: %
  IO_CAN_ReadMsg : IOBlock_Library_TTC580/CAN  Blocks TTC580 IOlib/ReadMsg_CAN/IO_CAN_ReadMsg  SampleTime=-1  ttlib=IO_Blk_Lib_TTC500  ttDescription=IO_CAN_ReadMsg  tt_iolib_version=0.19
      settings: SourceProductName=I/O Blocklibrary for TTC580
  Terminator{1..2,6..8} (5 alike) : Terminator
  ErrorCode : Outport  VectorParamsAs1DForOutWhenUnconnected=off
  wires:
  IO_CAN_ConfigMsg/1(ErrorCode) -> Terminator2/1
  IO_CAN_ConfigMsg/2(handle) -> IO_CAN_ReadMsg/1
  IO_CAN_ReadMsg/2 -> Terminator1/1
  IO_CAN_ReadMsg/1 -> ErrorCode/1
  IO_CAN_ReadMsg/5 -> Terminator6/1
  IO_CAN_ReadMsg/4 -> Terminator7/1
  IO_CAN_ReadMsg/3 -> Terminator8/1

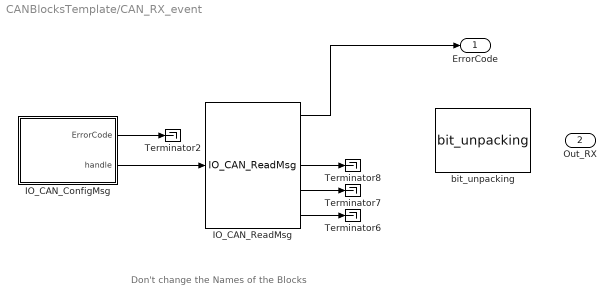
== system CANBlocksTemplate/CAN_RX_event ==
  note: Don't change the Names of the Blocks
  IO_CAN_ConfigMsg : Subsystem  mask(IO_CAN_ConfigMsg_Code){SampleTime=-1, ttlib=IO_Blk_Lib_TTC500, ttDescription=IO_CAN_ConfigMsg, tt_iolib_version=0.19, channel=IO_CAN_CHANNEL_0, mode=IO_CAN_MSG_READ, id_format=IO_CAN_STD_FRAME, id=0x1, ac_mask=0x7FF}
      mask help: Configures a message object for the given CAN channel.
      mask init:
      | %
      settings: CopyFcn=%deleted
      mask Help: web(which('IO_CAN.h'))
      mask TypeOptions channel: IO_CAN_CHANNEL_0  | IO_CAN_CHANNEL_1 | IO_CAN_CHANNEL_2 | IO_CAN_CHANNEL_3 | IO_CAN_CHANNEL_4 | IO_CAN_CHANNEL_5 | IO_CAN_CHANNEL_6
      mask Callback channel: %
      mask TypeOptions mode: IO_CAN_MSG_READ | IO_CAN_MSG_WRITE
      mask Callback mode: %
      mask TypeOptions id_format: IO_CAN_STD_FRAME | IO_CAN_EXT_FRAME
      mask Callback id_format: %
      mask Callback id: %
      mask Callback ac_mask: %
  IO_CAN_ReadMsg : IOBlock_Library_TTC580/CAN  Blocks TTC580 IOlib/ReadMsg_CAN/IO_CAN_ReadMsg  SampleTime=-1  ttlib=IO_Blk_Lib_TTC500  ttDescription=IO_CAN_ReadMsg  tt_iolib_version=0.19
      settings: SourceProductName=I/O Blocklibrary for TTC580
  Terminator{2,6..8} (4 alike) : Terminator
  bit_unpacking : IOBlock_Library_TTC580/CAN  Blocks TTC580 IOlib/bit_unpacking  SampleTime=-1  ttlib=IO_Blk_Lib_TTC500  ttDescription=bit_unpacking  tt_iolib_version=0.26  Endianness=little  Format=unsigned  Inversion=off  Startbit=0  Width_bits=8  Factor=1.0  Offset=0.0
      settings: SourceProductName=I/O Blocklibrary for TTC580
  ErrorCode : Outport  VectorParamsAs1DForOutWhenUnconnected=off
  Out_RX : Outport  Port=2  VectorParamsAs1DForOutWhenUnconnected=off
  wires:
  IO_CAN_ReadMsg/1 -> ErrorCode/1
  IO_CAN_ConfigMsg/1(ErrorCode) -> Terminator2/1
  IO_CAN_ConfigMsg/2(handle) -> IO_CAN_ReadMsg/1
  IO_CAN_ReadMsg/5 -> Terminator6/1
  IO_CAN_ReadMsg/4 -> Terminator7/1
  IO_CAN_ReadMsg/3 -> Terminator8/1

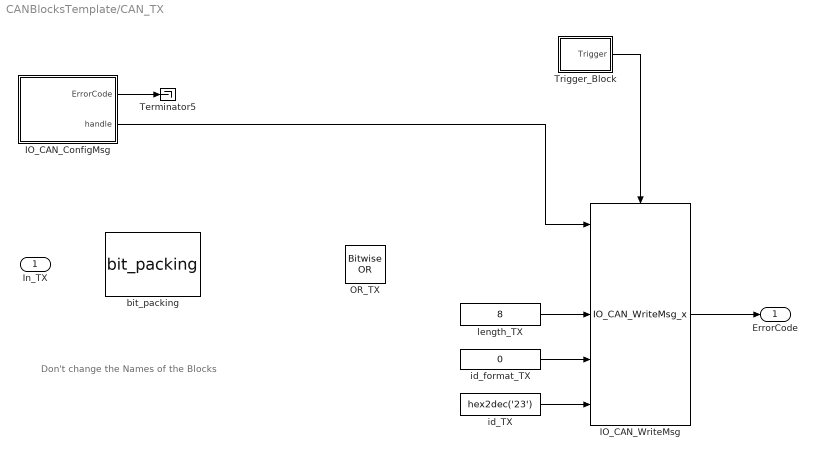
== system CANBlocksTemplate/CAN_TX ==
  note: Don't change the Names of the Blocks
  In_TX : Inport
  IO_CAN_ConfigMsg : Subsystem  mask(IO_CAN_ConfigMsg_Code){SampleTime=-1, ttlib=IO_Blk_Lib_TTC500, ttDescription=IO_CAN_ConfigMsg, tt_iolib_version=0.19, channel=IO_CAN_CHANNEL_0, mode=IO_CAN_MSG_READ, id_format=IO_CAN_STD_FRAME, id=0x1, ac_mask=0x7FF}
      mask help: Configures a message object for the given CAN channel.
      mask init:
      | %
      settings: CopyFcn=%deleted
      mask Help: web(which('IO_CAN.h'))
      mask TypeOptions channel: IO_CAN_CHANNEL_0  | IO_CAN_CHANNEL_1 | IO_CAN_CHANNEL_2 | IO_CAN_CHANNEL_3 | IO_CAN_CHANNEL_4 | IO_CAN_CHANNEL_5 | IO_CAN_CHANNEL_6
      mask Callback channel: %
      mask TypeOptions mode: IO_CAN_MSG_READ | IO_CAN_MSG_WRITE
      mask Callback mode: %
      mask TypeOptions id_format: IO_CAN_STD_FRAME | IO_CAN_EXT_FRAME
      mask Callback id_format: %
      mask Callback id: %
      mask Callback ac_mask: %
  IO_CAN_WriteMsg : IOBlock_Library_TTC580/CAN  Blocks TTC580 IOlib/WriteMsg_CAN_derated/IO_CAN_WriteMsg_x  SampleTime=-1  ttlib=IO_Blk_Lib_TTC500  ttDescription=IO_CAN_WriteMsg  tt_iolib_version=0.19
      settings: SourceProductName=I/O Blocklibrary for TTC580
  OR_TX : simulink/Logic and Bit Operations/Bitwise Operator  logicop=OR  UseBitMask=off  BitMask=bin2dec('11011001')  BitMaskRealWorld=Stored Integer
  Terminator5 : Terminator
  Trigger_Block : Subsystem  mask(Derate Trigger){derate=1, trigger_offset=0}
      mask prompts: trigger_offset "offset for the trigger"
      mask help: derate "n": every n-th cylce a trigger is submitted
  bit_packing : IOBlock_Library_TTC580/CAN  Blocks TTC580 IOlib/bit_packing  SampleTime=-1  ttlib=IO_Blk_Lib_TTC500  ttDescription=bit_packing  tt_iolib_version=0.26  Endianness=little  Format=unsigned  Inversion=off  Startbit=0  Width_bits=8  Factor=1.0  Offset=0.0
      settings: SourceProductName=I/O Blocklibrary for TTC580
  id_TX : Constant  Value=hex2dec('23')  OutDataTypeStr=uint32
  id_format_TX : Constant  Value=0  OutDataTypeStr=Inherit: Inherit via back propagation
  length_TX : Constant  Value=8  OutDataTypeStr=Inherit: Inherit via back propagation
  ErrorCode : Outport  VectorParamsAs1DForOutWhenUnconnected=off
  wires:
  id_TX/1 -> IO_CAN_WriteMsg/5
  id_format_TX/1 -> IO_CAN_WriteMsg/4
  length_TX/1 -> IO_CAN_WriteMsg/3
  IO_CAN_ConfigMsg/2(handle) -> IO_CAN_WriteMsg/1
  IO_CAN_ConfigMsg/1(ErrorCode) -> Terminator5/1
  IO_CAN_WriteMsg/1 -> ErrorCode/1
  Trigger_Block/1(Trigger) -> IO_CAN_WriteMsg/Enable

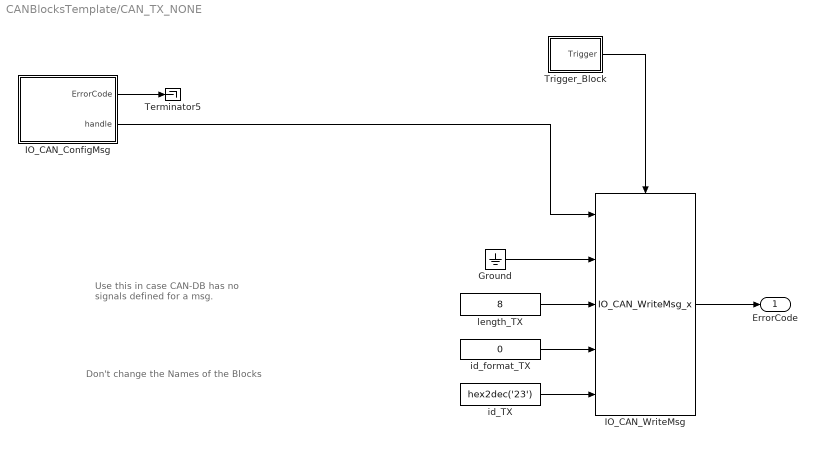
== system CANBlocksTemplate/CAN_TX_NONE ==
  note: Use this in case CAN-DB
      | has no signals defined for a msg.
  note: Don't change the Names of the Blocks
  Ground : Ground
  IO_CAN_ConfigMsg : Subsystem  mask(IO_CAN_ConfigMsg_Code){SampleTime=-1, ttlib=IO_Blk_Lib_TTC500, ttDescription=IO_CAN_ConfigMsg, tt_iolib_version=0.19, channel=IO_CAN_CHANNEL_0, mode=IO_CAN_MSG_READ, id_format=IO_CAN_STD_FRAME, id=0x1, ac_mask=0x7FF}
      mask help: Configures a message object for the given CAN channel.
      mask init:
      | %
      settings: CopyFcn=%deleted
      mask Help: web(which('IO_CAN.h'))
      mask TypeOptions channel: IO_CAN_CHANNEL_0  | IO_CAN_CHANNEL_1 | IO_CAN_CHANNEL_2 | IO_CAN_CHANNEL_3 | IO_CAN_CHANNEL_4 | IO_CAN_CHANNEL_5 | IO_CAN_CHANNEL_6
      mask Callback channel: %
      mask TypeOptions mode: IO_CAN_MSG_READ | IO_CAN_MSG_WRITE
      mask Callback mode: %
      mask TypeOptions id_format: IO_CAN_STD_FRAME | IO_CAN_EXT_FRAME
      mask Callback id_format: %
      mask Callback id: %
      mask Callback ac_mask: %
  IO_CAN_WriteMsg : IOBlock_Library_TTC580/CAN  Blocks TTC580 IOlib/WriteMsg_CAN_derated/IO_CAN_WriteMsg_x  SampleTime=-1  ttlib=IO_Blk_Lib_TTC500  ttDescription=IO_CAN_WriteMsg  tt_iolib_version=0.19
      settings: SourceProductName=I/O Blocklibrary for TTC580
  Terminator5 : Terminator
  Trigger_Block : Subsystem  mask(Derate Trigger){derate=1, trigger_offset=0}
      mask prompts: trigger_offset "offset for the trigger"
      mask help: derate "n": every n-th cylce a trigger is submitted
  id_TX : Constant  Value=hex2dec('23')  OutDataTypeStr=uint32
  id_format_TX : Constant  Value=0  OutDataTypeStr=Inherit: Inherit via back propagation
  length_TX : Constant  Value=8  OutDataTypeStr=Inherit: Inherit via back propagation
  ErrorCode : Outport  VectorParamsAs1DForOutWhenUnconnected=off
  wires:
  id_TX/1 -> IO_CAN_WriteMsg/5
  id_format_TX/1 -> IO_CAN_WriteMsg/4
  length_TX/1 -> IO_CAN_WriteMsg/3
  IO_CAN_WriteMsg/1 -> ErrorCode/1
  Ground/1 -> IO_CAN_WriteMsg/2
  Trigger_Block/1(Trigger) -> IO_CAN_WriteMsg/Enable
  IO_CAN_ConfigMsg/2(handle) -> IO_CAN_WriteMsg/1
  IO_CAN_ConfigMsg/1(ErrorCode) -> Terminator5/1

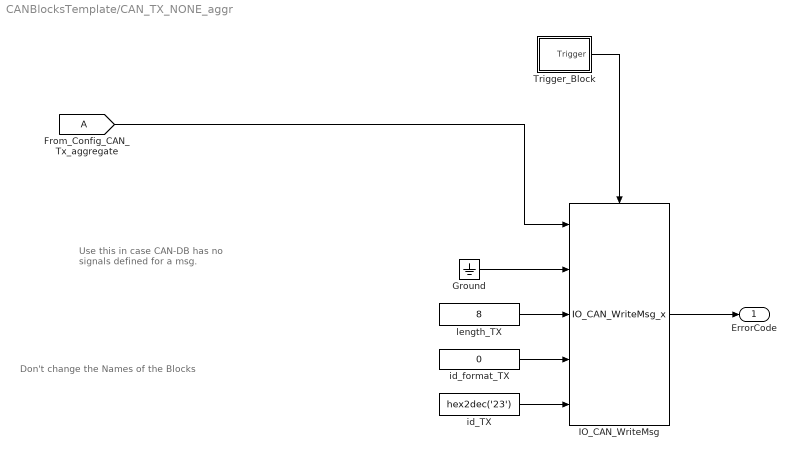
== system CANBlocksTemplate/CAN_TX_NONE_aggr ==
  note: Don't change the Names of the Blocks
  note: Use this in case CAN-DB
      | has no signals defined for a msg.
  Ground : Ground
  IO_CAN_WriteMsg : IOBlock_Library_TTC580/CAN  Blocks TTC580 IOlib/WriteMsg_CAN_derated/IO_CAN_WriteMsg_x  SampleTime=-1  ttlib=IO_Blk_Lib_TTC500  ttDescription=IO_CAN_WriteMsg  tt_iolib_version=0.19
      settings: SourceProductName=I/O Blocklibrary for TTC580
  Trigger_Block : Subsystem  mask(Derate Trigger){derate=1, trigger_offset=0}
      mask prompts: trigger_offset "offset for the trigger"
      mask help: derate "n": every n-th cylce a trigger is submitted
  id_TX : Constant  Value=hex2dec('23')  OutDataTypeStr=uint32
  id_format_TX : Constant  Value=0  OutDataTypeStr=Inherit: Inherit via back propagation
  length_TX : Constant  Value=8  OutDataTypeStr=Inherit: Inherit via back propagation
  ErrorCode : Outport  VectorParamsAs1DForOutWhenUnconnected=off
  wires:
  Trigger_Block/1(Trigger) -> IO_CAN_WriteMsg/Enable
  IO_CAN_WriteMsg/1 -> ErrorCode/1
  [A] -> IO_CAN_WriteMsg/1
  length_TX/1 -> IO_CAN_WriteMsg/3
  id_format_TX/1 -> IO_CAN_WriteMsg/4
  id_TX/1 -> IO_CAN_WriteMsg/5
  Ground/1 -> IO_CAN_WriteMsg/2

== system CANBlocksTemplate/CAN_TX_NONE_event ==
  note: Don't change the Names of the Blocks
  note: Use this in case CAN-DB
      | has no signals defined for a msg.
  Ground : Ground
  IO_CAN_ConfigMsg : Subsystem  mask(IO_CAN_ConfigMsg_Code){SampleTime=-1, ttlib=IO_Blk_Lib_TTC500, ttDescription=IO_CAN_ConfigMsg, tt_iolib_version=0.19, channel=IO_CAN_CHANNEL_0, mode=IO_CAN_MSG_READ, id_format=IO_CAN_STD_FRAME, id=0x1, ac_mask=0x7FF}
      mask help: Configures a message object for the given CAN channel.
      mask init:
      | %
      settings: CopyFcn=%deleted
      mask Help: web(which('IO_CAN.h'))
      mask TypeOptions channel: IO_CAN_CHANNEL_0  | IO_CAN_CHANNEL_1 | IO_CAN_CHANNEL_2 | IO_CAN_CHANNEL_3 | IO_CAN_CHANNEL_4 | IO_CAN_CHANNEL_5 | IO_CAN_CHANNEL_6
      mask Callback channel: %
      mask TypeOptions mode: IO_CAN_MSG_READ | IO_CAN_MSG_WRITE
      mask Callback mode: %
      mask TypeOptions id_format: IO_CAN_STD_FRAME | IO_CAN_EXT_FRAME
      mask Callback id_format: %
      mask Callback id: %
      mask Callback ac_mask: %
  IO_CAN_WriteMsg : IOBlock_Library_TTC580/CAN  Blocks TTC580 IOlib/WriteMsg_CAN/IO_CAN_WriteMsg  SampleTime=-1  ttlib=IO_Blk_Lib_TTC500  ttDescription=IO_CAN_WriteMsg  tt_iolib_version=0.19
      settings: SourceProductName=I/O Blocklibrary for TTC580
  Terminator5 : Terminator
  id_TX : Constant  Value=hex2dec('23')  OutDataTypeStr=uint32
  id_format_TX : Constant  Value=0  OutDataTypeStr=Inherit: Inherit via back propagation
  length_TX : Constant  Value=8  OutDataTypeStr=Inherit: Inherit via back propagation
  ErrorCode : Outport  VectorParamsAs1DForOutWhenUnconnected=off
  wires:
  IO_CAN_ConfigMsg/1(ErrorCode) -> Terminator5/1
  IO_CAN_ConfigMsg/2(handle) -> IO_CAN_WriteMsg/1
  Ground/1 -> IO_CAN_WriteMsg/2
  IO_CAN_WriteMsg/1 -> ErrorCode/1
  length_TX/1 -> IO_CAN_WriteMsg/3
  id_format_TX/1 -> IO_CAN_WriteMsg/4
  id_TX/1 -> IO_CAN_WriteMsg/5

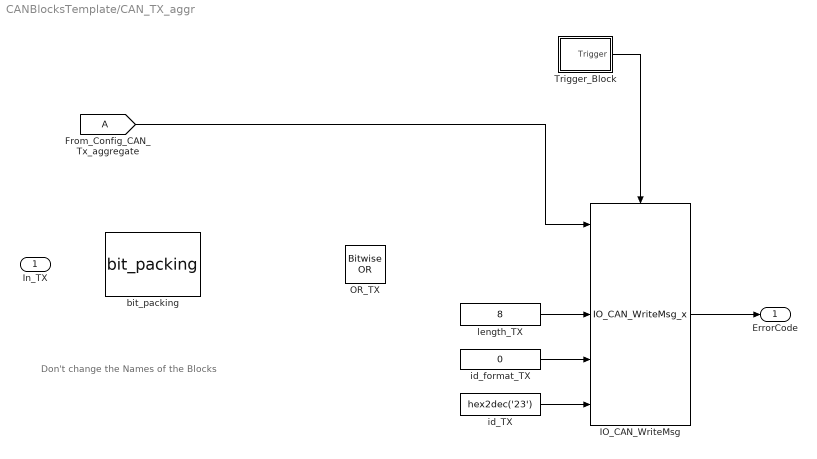
== system CANBlocksTemplate/CAN_TX_aggr ==
  note: Don't change the Names of the Blocks
  In_TX : Inport
  IO_CAN_WriteMsg : IOBlock_Library_TTC580/CAN  Blocks TTC580 IOlib/WriteMsg_CAN_derated/IO_CAN_WriteMsg_x  SampleTime=-1  ttlib=IO_Blk_Lib_TTC500  ttDescription=IO_CAN_WriteMsg  tt_iolib_version=0.19
      settings: SourceProductName=I/O Blocklibrary for TTC580
  OR_TX : simulink/Logic and Bit Operations/Bitwise Operator  logicop=OR  UseBitMask=off  BitMask=bin2dec('11011001')  BitMaskRealWorld=Stored Integer
  Trigger_Block : Subsystem  mask(Derate Trigger){derate=1, trigger_offset=0}
      mask prompts: trigger_offset "offset for the trigger"
      mask help: derate "n": every n-th cylce a trigger is submitted
  bit_packing : IOBlock_Library_TTC580/CAN  Blocks TTC580 IOlib/bit_packing  SampleTime=-1  ttlib=IO_Blk_Lib_TTC500  ttDescription=bit_packing  tt_iolib_version=0.26  Endianness=little  Format=unsigned  Inversion=off  Startbit=0  Width_bits=8  Factor=1.0  Offset=0.0
      settings: SourceProductName=I/O Blocklibrary for TTC580
  id_TX : Constant  Value=hex2dec('23')  OutDataTypeStr=uint32
  id_format_TX : Constant  Value=0  OutDataTypeStr=Inherit: Inherit via back propagation
  length_TX : Constant  Value=8  OutDataTypeStr=Inherit: Inherit via back propagation
  ErrorCode : Outport  VectorParamsAs1DForOutWhenUnconnected=off
  wires:
  id_TX/1 -> IO_CAN_WriteMsg/5
  id_format_TX/1 -> IO_CAN_WriteMsg/4
  length_TX/1 -> IO_CAN_WriteMsg/3
  [A] -> IO_CAN_WriteMsg/1
  IO_CAN_WriteMsg/1 -> ErrorCode/1
  Trigger_Block/1(Trigger) -> IO_CAN_WriteMsg/Enable
